simulink model "rc_ckt"  (R2020a)
settings: Solver=VariableStepAuto  StartTime=0.0  StopTime=10.0  RelTol=1e-3
settings Model: Creator=kolep  LastModifiedBy=kolep

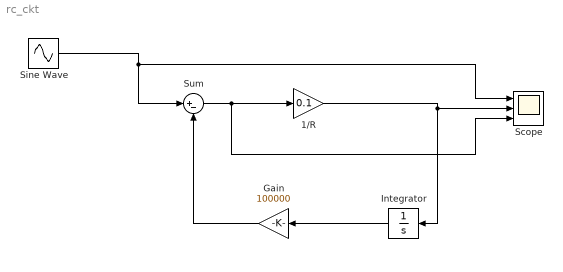
== system rc_ckt ==
  1/R : Gain  Gain=0.1
  Gain : Gain  Gain=100000
  Integrator : Integrator
  Scope : Scope  NumInputPorts=3
  Sine Wave : Sin  SampleTime=0
  Sum : Sum  Inputs=|+-
  wires:
  Sine Wave/1 -> Sum/1, Scope/1
  Sum/1 -> Scope/3, 1/R/1
  1/R/1 -> Integrator/1, Scope/2
  Integrator/1 -> Gain/1
  Gain/1 -> Sum/2
